simulink model "DPLL_2ndType_2rdOrder_model"  (R2016a)
settings: Solver=ode45  StartTime=0  StopTime=80e-6  FixedStep=100e-12  MaxStep=1e-10  RelTol=1e-6  AbsTol=1e-12
values from neighbouring files (symbols this model uses):
  a = 4.7848e8    (= 478480000)    [DPLL_2ndType_2ndOrder.m]
  b = 1.7776e-4    (= 0.00017776)    [DPLL_2ndType_2ndOrder.m]
  c = 2.167e7    (= 21670000)    [DPLL_2ndType_2ndOrder.m]
  d = 1.735e-3    (= 0.001735)    [DPLL_2ndType_2ndOrder.m]
  fref_num = 1/13e-9    (= 76923076.9231)    [DPLL_2ndType_2ndOrder.m]    (also in test.m = 200000000)
  Ki_num = 2^-4    (= 0.0625)    [DPLL_2ndType_2ndOrder.m]    (also in test.m = 0.00390625)
  Kp_num = 5    [DPLL_2ndType_2ndOrder.m]    (also in test.m = 0.75)
  N_num = 10    [DPLL_2ndType_2ndOrder.m]    (also in MDLL.m = 16; PLL_2ndType_2ndOrder.m = 8; PLL_2ndType_3rdOrder.m = 56; test.m = 20)
undefined symbols (not defined in the file): Kv_num
libraries: simulink_extras x3, dspswit3 x1
settings Model: SimulationMode=accelerator  Creator=asus  LastModifiedBy=xzhang
settings SolverCC: ShapePreserveControl=EnableAll  ZeroCrossControl=EnableAll  ZeroCrossAlgorithm=Adaptive
settings DataIOCC: LimitDataPoints=on  SaveFormat=Array  SignalLoggingSaveFormat=ModelDataLogs
settings OptimizationCC: ExpressionDepthLimit=2147483647  EfficientMapNaN2IntZero=off  SimCompilerOptimization=on
settings DebuggingCC: UnderspecifiedInitializationDetection=Classic  MergeDetectMultiDrivingBlocksExec=none  SolverPrmCheckMsg=warning  FcnCallInpInsideContextMsg=EnableAllAsWarning  AllowSymbolicDim=off  StateNameClashWarn=warning
settings HardwareCC: ProdBitPerPointer=32  ProdLargestAtomicFloat=None  ProdIntDivRoundTo=Undefined  ProdEndianess=Unspecified  ProdWordSize=32  ProdHWDeviceType=32-bit Generic  TargetBitPerPointer=64  TargetLongLongMode=on  TargetIntDivRoundTo=Zero  TargetEndianess=LittleEndian  TargetWordSize=64  TargetHWDeviceType=MATLAB Host  ProdEqTarget=off
settings ModelReferenceCC: PropagateSignalLabelsOutOfModel=off
settings CodeAppCC: MaxIdLength=128
settings GRTTargetCC: GeneratePreprocessorConditionals=Use local settings  CombineOutputUpdateFcns=off  GRTInterface=on
settings ConfigComp: CovModelRefEnable=Off
settings ConfigurationSet: Description=SimMechanics 2G

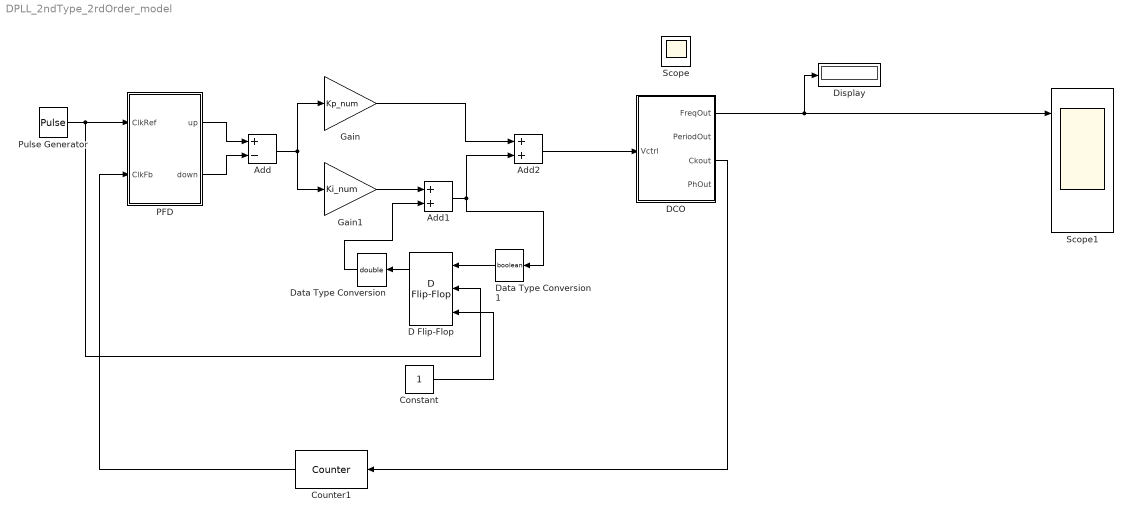
== system DPLL_2ndType_2rdOrder_model ==
  Add : Sum  Inputs=+-
  Add1 : Sum  AccumDataTypeStr=fixdt(1,16,2^0,0)
  Add2 : Sum
  Constant : Constant
  Counter1 : dspswit3/Counter  Direction=Up  CountEvent=Rising edge  CounterSize=User defined  MaxCount=N_num-1  InitialCount=0  Output=Hit  HitValue=N_num-1  ResetInput=off  SamplesPerFrame=1  Ts=1  CntDtype=double  HitDtype=Logical
  D Flip-Flop : simulink_extras/Flip Flops/D Flip-Flop
  DCO : Subsystem  mask{f0=0, Kvco=Kv_num}
      mask prompts: f0 "Free Running Freq.(Hz)"; Kvco "VCO Gain(Hz/V)"
  Data Type Conversion : DataTypeConversion  OutDataTypeStr=double
  Data Type Conversion1 : DataTypeConversion  OutDataTypeStr=boolean
  Display : Display
      settings: Format=short_e  Decimation=N_num
  Gain : Gain  Gain=Kp_num
  Gain1 : Gain  Gain=Ki_num
  PFD : Subsystem
  Pulse Generator : DiscretePulseGenerator  PulseType=Time based  Period=1/fref_num  PulseWidth=50  SampleTime=1/fref_num/10
  Scope : Scope
  Scope1 : Scope  NumInputPorts=3
  wires:
  Pulse Generator/1 -> D Flip-Flop/2, PFD/1(ClkRef)
  DCO/1(FreqOut) -> Scope1/1, Display/1
  Counter1/1 -> PFD/2(ClkFb)
  DCO/3(Ckout) -> Counter1/1
  PFD/2(down) -> Add/2
  PFD/1(up) -> Add/1
  Gain/1 -> Add2/1
  Add/1 -> Gain1/1, Gain/1
  Gain1/1 -> Add1/1
  Add1/1 -> Data Type Conversion1/1, Add2/2
  Add2/1 -> DCO/1(Vctrl)
  Constant/1 -> D Flip-Flop/3
  D Flip-Flop/1 -> Data Type Conversion/1
  Data Type Conversion/1 -> Add1/2
  Data Type Conversion1/1 -> D Flip-Flop/1

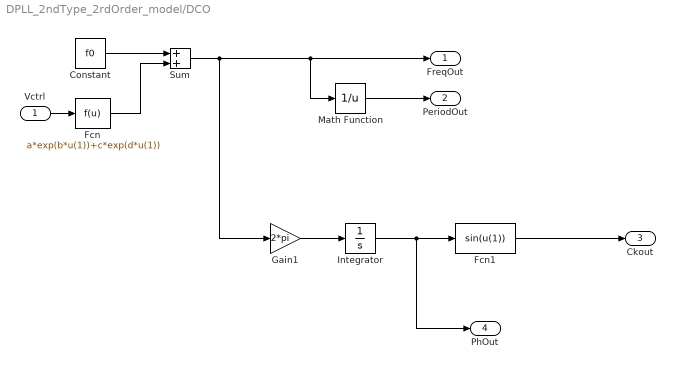
== system DPLL_2ndType_2rdOrder_model/DCO ==
  Vctrl : Inport
  Constant : Constant  Value=f0
  Fcn : Fcn  Expr=a*exp(b*u(1))+c*exp(d*u(1))
  Fcn1 : Fcn  Expr=sin(u(1))
  Gain1 : Gain  Gain=2*pi
  Integrator : Integrator
  Math Function : Math  Operator=reciprocal  SaturateOnIntegerOverflow=on
  Sum : Sum
  FreqOut : Outport
  PeriodOut : Outport  Port=2
  Ckout : Outport  Port=3
  PhOut : Outport  Port=4
  wires:
  Constant/1 -> Sum/1
  Fcn/1 -> Sum/2
  Sum/1 -> Gain1/1, FreqOut/1, Math Function/1
  Vctrl/1 -> Fcn/1
  Fcn1/1 -> Ckout/1
  Integrator/1 -> PhOut/1, Fcn1/1
  Gain1/1 -> Integrator/1
  Math Function/1 -> PeriodOut/1

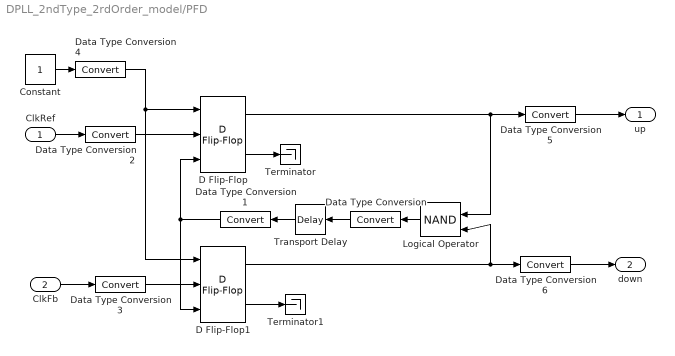
== system DPLL_2ndType_2rdOrder_model/PFD ==
  ClkRef : Inport
  ClkFb : Inport  Port=2
  Constant : Constant
  D Flip-Flop : simulink_extras/Flip Flops/D Flip-Flop
  D Flip-Flop1 : simulink_extras/Flip Flops/D Flip-Flop
  Data Type Conversion{,1..6} (7 alike) : DataTypeConversion
  Logical Operator : Logic  Operator=NAND  IconShape=distinctive  AllPortsSameDT=off  OutDataTypeStr=boolean
  Terminator : Terminator
  Terminator1 : Terminator
  Transport Delay : TransportDelay  DelayTime=200e-12  BufferSize=2048
  up : Outport
  down : Outport  Port=2
  wires:
  D Flip-Flop/1 -> Logical Operator/1, Data Type Conversion5/1
  D Flip-Flop1/1 -> Logical Operator/2, Data Type Conversion6/1
  Constant/1 -> Data Type Conversion4/1
  ClkRef/1 -> Data Type Conversion2/1
  ClkFb/1 -> Data Type Conversion3/1
  Data Type Conversion/1 -> Transport Delay/1
  Transport Delay/1 -> Data Type Conversion1/1
  Logical Operator/1 -> Data Type Conversion/1
  Data Type Conversion1/1 -> D Flip-Flop1/3, D Flip-Flop/3
  D Flip-Flop/2 -> Terminator/1
  D Flip-Flop1/2 -> Terminator1/1
  Data Type Conversion2/1 -> D Flip-Flop/2
  Data Type Conversion3/1 -> D Flip-Flop1/2
  Data Type Conversion4/1 -> D Flip-Flop/1, D Flip-Flop1/1
  Data Type Conversion5/1 -> up/1
  Data Type Conversion6/1 -> down/1
